simulink model "s2eig"  (Simulink 2.00)
settings: Solver=ode45  StartTime=0.0  StopTime=tstop  MaxStep=0.04  RelTol=1e-6  AbsTol=1e-6
values from neighbouring files (symbols this model uses):
  AEx = 0.0012    [I3ESSR.M]    (also in SET1.M)
  BEx = 1.264    [I3ESSR.M]    (also in SET1.M)
  delio = x(3)    [M1.M]    (also in M3.M = delta4; M3G.M = delta4; M4.M = delta)
  Domega = 0    [I3ESSR.M]    (also in M3.M; M3G.M; M5.M = 1; SET1.M = 2)
  Edpo = x(2)    [M1.M]    (also in M4.M = Vdo - xpq*Iqo + rs*Ido)
  Eqpo = x(1)    [M1.M]    (also in M4.M = Vqo + xpd*Ido + rs*Iqo)
  H = 2.89    [I3ESSR.M]    (also in M1.M = 0.5*J_rotor*wbasem*wbasem/Sbase; M3.M = diag(h); M3G.M = diag(h); M5.M = 0.352825293175)
  KA = 50    [I3ESSR.M]    (also in SET1.M)
  KE = -0.0465    [I3ESSR.M]    (also in SET1.M)
  KF = 0.0832    [I3ESSR.M]    (also in SET1.M)
  rs = 0.00    (= 0)    [I3ESSR.M]    (also in M1.M = rs/Zbase; M3.M; M3G.M = 0.001; M5.M = rs/Zb)
  TA = .06    (= 0.06)    [I3ESSR.M]    (also in SET1.M)
  TE = 0.052    [I3ESSR.M]    (also in SET1.M)
  TF = 1.0    (= 1)    [I3ESSR.M]    (also in SET1.M)
  Tpdo = 4.3    [I3ESSR.M]    (also in SET1.M = 7.9)
  Tpqo = 0.85    [I3ESSR.M]    (also in SET1.M = 0.41)
  VR = KE*Efo    [M4.M]
  VRmax = 1    [I3ESSR.M]    (also in SET1.M)
  VRmin = -1    [I3ESSR.M]    (also in SET1.M)
  Vs = Efo*KF/TF    [M4.M]
  wb = wbase    [M1.M]    (also in M2.M = 376.991118431; M3.M = 376.991118431; M3G.M = 376.991118431; M4.M = we)
  xd = 1.79    [I3ESSR.M]    (also in M1.M = xd/Zbase; M3.M; M3G.M; M5.M = xd/Zb)
  xpd = 0.169    [I3ESSR.M]    (also in M1.M = xpd/Zbase; SET1.M = 0.355)
  xq = 1.71    [I3ESSR.M]    (also in M1.M = xq/Zbase; M3.M; M3G.M; M5.M = xq/Zb)
undefined symbols (not defined in the file or in its folder): Ef, Exc_sw, Sbratio
settings Model: SaveTime=off  SaveOutput=off  ConsistencyChecking=off

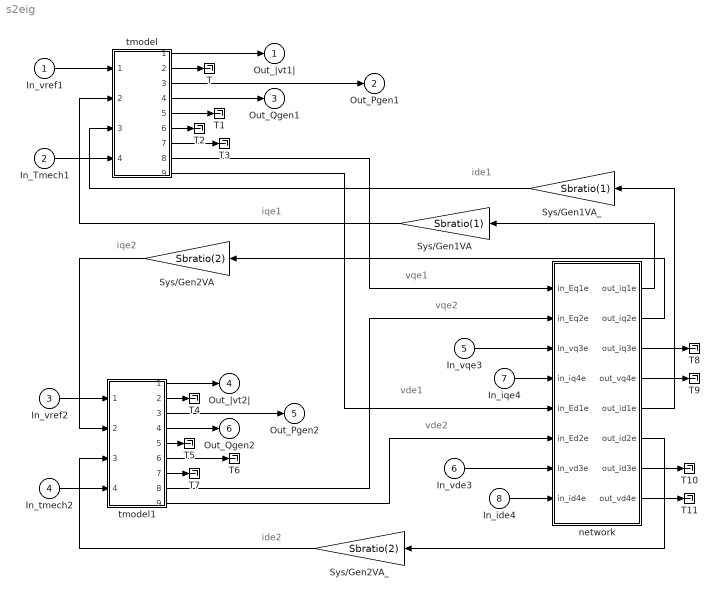
== system s2eig ==
  note: vqe1
  note: vqe2
  note: vde1
  note: vde2
  note: iqe2
  note: ide1
  note: iqe1
  note: ide2
  In_vref1 : Inport  Port=1  PortWidth=-1  SampleTime=-1
  In_Tmech1 : Inport  Port=2  PortWidth=-1  SampleTime=-1
  In_vref2 : Inport  Port=3  PortWidth=-1  SampleTime=-1
  In_tmech2 : Inport  Port=4  PortWidth=-1  SampleTime=-1
  In_vqe3 : Inport  Port=5  PortWidth=-1  SampleTime=-1
  In_vde3 : Inport  Port=6  PortWidth=-1  SampleTime=-1
  In_iqe4 : Inport  Port=7  PortWidth=-1  SampleTime=-1
  In_ide4 : Inport  Port=8  PortWidth=-1  SampleTime=-1
  Sys/Gen1VA : Gain  Orientation=left  Gain=Sbratio(1)
  Sys/Gen1VA_ : Gain  Orientation=left  Gain=Sbratio(1)
  Sys/Gen2VA : Gain  Orientation=left  Gain=Sbratio(2)
  Sys/Gen2VA_ : Gain  Orientation=left  Gain=Sbratio(2)
  T{,1..11} (12 alike) : Terminator
  network : Subsystem
  tmodel : Subsystem
  tmodel1 : Subsystem
  Out_|vt1| : Outport  Port=1  InitialOutput=0
  Out_Pgen1 : Outport  Port=2  InitialOutput=0
  Out_Qgen1 : Outport  Port=3  InitialOutput=0
  Out_|vt2| : Outport  Port=4  InitialOutput=0
  Out_Pgen2 : Outport  Port=5  InitialOutput=0
  Out_Qgen2 : Outport  Port=6  InitialOutput=0
  wires:
  network/4(out_vq4e) -> T9/1
  network/3(out_iq3e) -> T8/1
  network/8(out_vd4e) -> T11/1
  network/7(out_id3e) -> T10/1
  tmodel1/7(out_Tem) -> T7/1
  tmodel1/6(out_puslip) -> T6/1
  tmodel1/5(out_delta) -> T5/1
  tmodel1/2(out_|I|) -> T4/1
  tmodel/7(out_Tem) -> T3/1
  tmodel/6(out_puslip) -> T2/1
  tmodel/5(out_delta) -> T1/1
  tmodel/2(out_|I|) -> T/1
  Sys/Gen1VA/1 -> tmodel/2(in_iqe)
  network/1(out_iq1e) -> Sys/Gen1VA/1
  Sys/Gen1VA_/1 -> tmodel/3(in_ide)
  network/5(out_id1e) -> Sys/Gen1VA_/1
  Sys/Gen2VA_/1 -> tmodel1/3(in_ide)
  network/6(out_id2e) -> Sys/Gen2VA_/1
  Sys/Gen2VA/1 -> tmodel1/2(in_iqe)
  network/2(out_iq2e) -> Sys/Gen2VA/1
  tmodel1/4(out_Qgen) -> Out_Qgen2/1
  tmodel1/3(out_Pgen) -> Out_Pgen2/1
  tmodel1/1(out_|Vt|) -> Out_|vt2|/1
  tmodel/4(out_Qgen) -> Out_Qgen1/1
  tmodel/3(out_Pgen) -> Out_Pgen1/1
  tmodel/1(out_|Vt|) -> Out_|vt1|/1
  In_ide4/1 -> network/8(in_id4e)
  In_iqe4/1 -> network/4(in_iq4e)
  In_vde3/1 -> network/7(in_vd3e)
  In_vqe3/1 -> network/3(in_vq3e)
  In_tmech2/1 -> tmodel1/4(in_Tmech)
  In_vref2/1 -> tmodel1/1(in_Vref)
  In_Tmech1/1 -> tmodel/4(in_Tmech)
  In_vref1/1 -> tmodel/1(in_Vref)
  tmodel1/9(out_Edpe) -> network/6(in_Ed2e)
  tmodel/9(out_Edpe) -> network/5(in_Ed1e)
  tmodel1/8(out_Eqpe) -> network/2(in_Eq2e)
  tmodel/8(out_Eqpe) -> network/1(in_Eq1e)

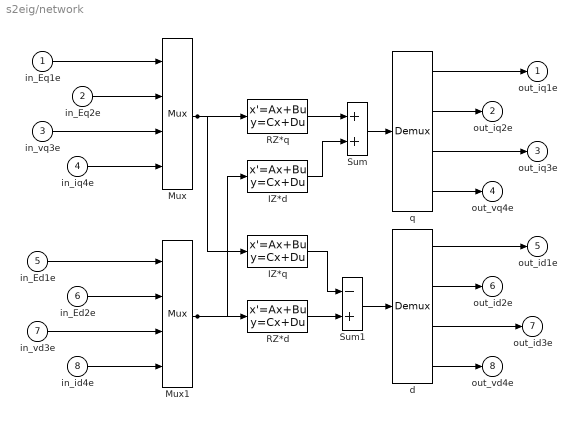
== system s2eig/network ==
  in_Eq1e : Inport  Port=1  PortWidth=-1  SampleTime=-1
  in_Eq2e : Inport  Port=2  PortWidth=-1  SampleTime=-1
  in_vq3e : Inport  Port=3  PortWidth=-1  SampleTime=-1
  in_iq4e : Inport  Port=4  PortWidth=-1  SampleTime=-1
  in_Ed1e : Inport  Port=5  PortWidth=-1  SampleTime=-1
  in_Ed2e : Inport  Port=6  PortWidth=-1  SampleTime=-1
  in_vd3e : Inport  Port=7  PortWidth=-1  SampleTime=-1
  in_id4e : Inport  Port=8  PortWidth=-1  SampleTime=-1
  IZ*d : StateSpace  A=[]  B=[]  C=[]  D=K  X0=0  mask(Matrix Gain){@1=IZ}
      mask prompts: @1 "Gain matrix:"
      mask help: Matrix Gain.
      mask init:
      | K = @1;
      mask Help: Multiplies input vector by entered matrix to produce output vector (y=Au).
      mask Display: disp('K')
  IZ*q : StateSpace  A=[]  B=[]  C=[]  D=K  X0=0  mask(Matrix Gain){@1=IZ}
      mask prompts: @1 "Gain matrix:"
      mask help: Matrix Gain.
      mask init:
      | K = @1;
      mask Help: Multiplies input vector by entered matrix to produce output vector (y=Au).
      mask Display: disp('K')
  Mux : Mux  Inputs=4
  Mux1 : Mux  Inputs=4
  RZ*d : StateSpace  A=[]  B=[]  C=[]  D=K  X0=0  mask(Matrix Gain){@1=RZ}
      mask prompts: @1 "Gain matrix:"
      mask help: Matrix Gain.
      mask init:
      | K = @1;
      mask Help: Multiplies input vector by entered matrix to produce output vector (y=Au).
      mask Display: disp('K')
  RZ*q : StateSpace  A=[]  B=[]  C=[]  D=K  X0=0  mask(Matrix Gain){@1=RZ}
      mask prompts: @1 "Gain matrix:"
      mask help: Matrix Gain.
      mask init:
      | K = @1;
      mask Help: Multiplies input vector by entered matrix to produce output vector (y=Au).
      mask Display: disp('K')
  Sum : Sum  Inputs=++
  Sum1 : Sum  Inputs=-+
  d : Demux  Outputs=4
  q : Demux  Outputs=4
  out_iq1e : Outport  Port=1  InitialOutput=0
  out_iq2e : Outport  Port=2  InitialOutput=0
  out_iq3e : Outport  Port=3  InitialOutput=0
  out_vq4e : Outport  Port=4  InitialOutput=0
  out_id1e : Outport  Port=5  InitialOutput=0
  out_id2e : Outport  Port=6  InitialOutput=0
  out_id3e : Outport  Port=7  InitialOutput=0
  out_vd4e : Outport  Port=8  InitialOutput=0
  wires:
  in_id4e/1 -> Mux1/4
  in_vd3e/1 -> Mux1/3
  in_Ed2e/1 -> Mux1/2
  in_Ed1e/1 -> Mux1/1
  in_iq4e/1 -> Mux/4
  in_vq3e/1 -> Mux/3
  in_Eq1e/1 -> Mux/1
  d/2 -> out_id2e/1
  d/4 -> out_vd4e/1
  d/3 -> out_id3e/1
  d/1 -> out_id1e/1
  q/2 -> out_iq2e/1
  in_Eq2e/1 -> Mux/2
  q/4 -> out_vq4e/1
  q/3 -> out_iq3e/1
  q/1 -> out_iq1e/1
  Mux/1 -> RZ*q/1, IZ*q/1
  Mux1/1 -> IZ*d/1, RZ*d/1
  RZ*q/1 -> Sum/1
  IZ*d/1 -> Sum/2
  IZ*q/1 -> Sum1/1
  RZ*d/1 -> Sum1/2
  Sum/1 -> q/1
  Sum1/1 -> d/1

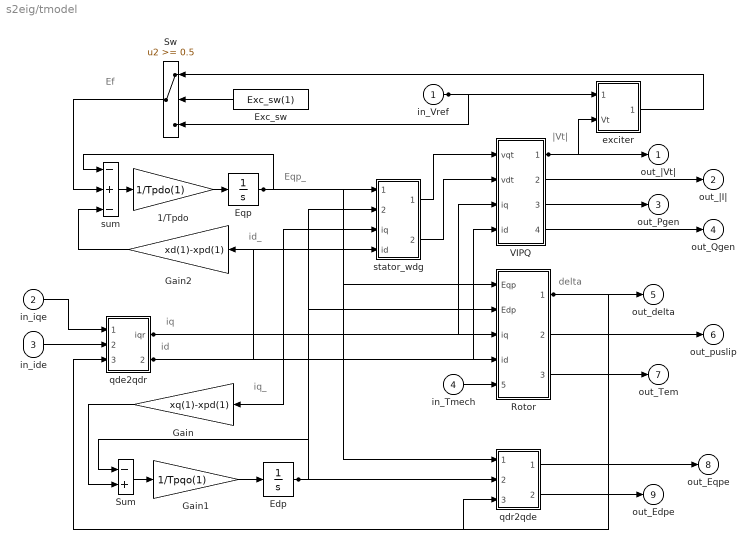
== system s2eig/tmodel ==
  note: iq_
  note: Ef
  note: delta
  note: id
  note: iq
  note: id_
  note: |Vt|
  note: Eqp_
  in_Vref : Inport  Port=1  PortWidth=-1  SampleTime=-1
  in_iqe : Inport  Port=2  PortWidth=-1  SampleTime=-1
  in_ide : Inport  Port=3  PortWidth=-1  SampleTime=-1
  in_Tmech : Inport  Port=4  PortWidth=-1  SampleTime=-1
  1/Tpdo : Gain  Gain=1/Tpdo(1)
  Edp : Integrator  ExternalReset=none  InitialConditionSource=internal  InitialCondition=Edpo(1)  LimitOutput=off  UpperSaturationLimit=inf  LowerSaturationLimit=-inf  ShowSaturationPort=off  ShowStatePort=off  AbsoluteTolerance=auto
  Eqp : Integrator  ExternalReset=none  InitialConditionSource=internal  InitialCondition=Eqpo(1)  LimitOutput=off  UpperSaturationLimit=inf  LowerSaturationLimit=-inf  ShowSaturationPort=off  ShowStatePort=off  AbsoluteTolerance=auto
  Exc_sw : Constant  Orientation=left  Value=Exc_sw(1)
  Gain : Gain  Orientation=left  Gain=xq(1)-xpd(1)
  Gain1 : Gain  Gain=1/Tpqo(1)
  Gain2 : Gain  Orientation=left  Gain=xd(1)-xpd(1)
  Rotor : Subsystem
  Sum : Sum  Inputs=-+
  Sw : Switch  Orientation=left  Threshold=0.5
  VIPQ : Subsystem
  exciter : Subsystem
  qde2qdr : Subsystem
  qdr2qde : Subsystem
  stator_wdg : Subsystem
  sum : Sum  Inputs=-+-
  out_|Vt| : Outport  Port=1  InitialOutput=0
  out_|I| : Outport  Port=2  InitialOutput=0
  out_Pgen : Outport  Port=3  InitialOutput=0
  out_Qgen : Outport  Port=4  InitialOutput=0
  out_delta : Outport  Port=5  InitialOutput=0
  out_puslip : Outport  Port=6  InitialOutput=0
  out_Tem : Outport  Port=7  InitialOutput=0
  out_Eqpe : Outport  Port=8  InitialOutput=0
  out_Edpe : Outport  Port=9  InitialOutput=0
  wires:
  in_Vref/1 -> Sw/3, exciter/1(Vref)
  stator_wdg/2(out_vdt) -> VIPQ/2(vdt)
  in_ide/1 -> qde2qdr/2(ide)
  qde2qdr/2(vdr) -> VIPQ/4(id), stator_wdg/4(id), Rotor/4(id), Gain2/1
  qde2qdr/1(iqr) -> VIPQ/3(iq), stator_wdg/3(iq), Rotor/3(iq), Gain/1
  Gain1/1 -> Edp/1
  Sum/1 -> Gain1/1
  Edp/1 -> qdr2qde/2(Edp), stator_wdg/2(Edp), Rotor/2(Edp), Sum/1
  Gain/1 -> Sum/2
  in_Tmech/1 -> Rotor/5(T_mech)
  qdr2qde/2(Edpe) -> out_Edpe/1
  qdr2qde/1(Eqpe) -> out_Eqpe/1
  VIPQ/1(out_|Vt|) -> out_|Vt|/1, exciter/2(Vt)
  stator_wdg/1(out_vqt) -> VIPQ/1(vqt)
  Rotor/3(Tem) -> out_Tem/1
  in_iqe/1 -> qde2qdr/1(iqe)
  Rotor/2(out_puslip) -> out_puslip/1
  Rotor/1(out_delta) -> qdr2qde/3(delta), out_delta/1, qde2qdr/3("delta ")
  VIPQ/4(out_Q) -> out_Qgen/1
  VIPQ/3(out_P) -> out_Pgen/1
  VIPQ/2(out_|I|) -> out_|I|/1
  Sw/1 -> sum/2
  Exc_sw/1 -> Sw/2
  exciter/1(out_Ef) -> Sw/1
  Gain2/1 -> sum/3
  sum/1 -> 1/Tpdo/1
  1/Tpdo/1 -> Eqp/1
  Eqp/1 -> qdr2qde/1(Eqp), sum/1, Rotor/1(Eqp), stator_wdg/1(Eqp)

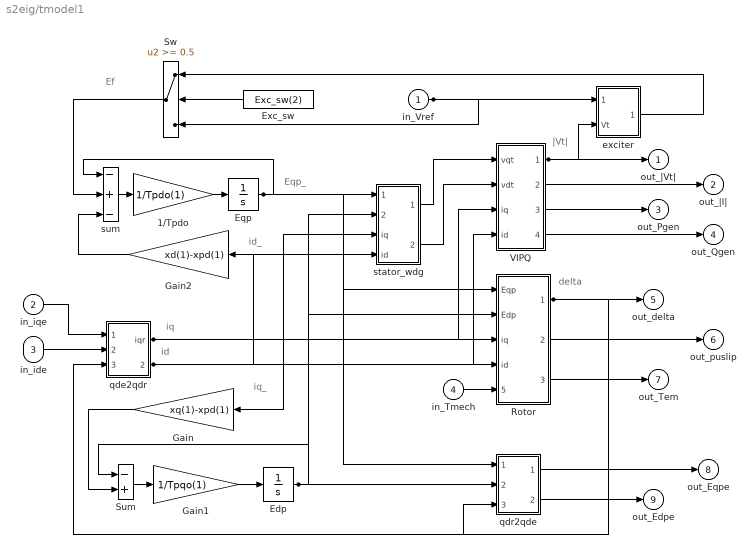
== system s2eig/tmodel1 ==
  note: id
  note: iq
  note: id_
  note: iq_
  note: delta
  note: Ef
  note: |Vt|
  note: Eqp_
  in_Vref : Inport  Port=1  PortWidth=-1  SampleTime=-1
  in_iqe : Inport  Port=2  PortWidth=-1  SampleTime=-1
  in_ide : Inport  Port=3  PortWidth=-1  SampleTime=-1
  in_Tmech : Inport  Port=4  PortWidth=-1  SampleTime=-1
  1/Tpdo : Gain  Gain=1/Tpdo(1)
  Edp : Integrator  ExternalReset=none  InitialConditionSource=internal  InitialCondition=Edpo(1)  LimitOutput=off  UpperSaturationLimit=inf  LowerSaturationLimit=-inf  ShowSaturationPort=off  ShowStatePort=off  AbsoluteTolerance=auto
  Eqp : Integrator  ExternalReset=none  InitialConditionSource=internal  InitialCondition=Eqpo(1)  LimitOutput=off  UpperSaturationLimit=inf  LowerSaturationLimit=-inf  ShowSaturationPort=off  ShowStatePort=off  AbsoluteTolerance=auto
  Exc_sw : Constant  Orientation=left  Value=Exc_sw(2)
  Gain : Gain  Orientation=left  Gain=xq(1)-xpd(1)
  Gain1 : Gain  Gain=1/Tpqo(1)
  Gain2 : Gain  Orientation=left  Gain=xd(1)-xpd(1)
  Rotor : Subsystem
  Sum : Sum  Inputs=-+
  Sw : Switch  Orientation=left  Threshold=0.5
  VIPQ : Subsystem
  exciter : Subsystem
  qde2qdr : Subsystem
  qdr2qde : Subsystem
  stator_wdg : Subsystem
  sum : Sum  Inputs=-+-
  out_|Vt| : Outport  Port=1  InitialOutput=0
  out_|I| : Outport  Port=2  InitialOutput=0
  out_Pgen : Outport  Port=3  InitialOutput=0
  out_Qgen : Outport  Port=4  InitialOutput=0
  out_delta : Outport  Port=5  InitialOutput=0
  out_puslip : Outport  Port=6  InitialOutput=0
  out_Tem : Outport  Port=7  InitialOutput=0
  out_Eqpe : Outport  Port=8  InitialOutput=0
  out_Edpe : Outport  Port=9  InitialOutput=0
  wires:
  in_Vref/1 -> Sw/3, exciter/1(Vref)
  stator_wdg/2(out_vdt) -> VIPQ/2(vdt)
  in_ide/1 -> qde2qdr/2(ide)
  qde2qdr/2(vdr) -> VIPQ/4(id), stator_wdg/4(id), Rotor/4(id), Gain2/1
  qde2qdr/1(iqr) -> VIPQ/3(iq), stator_wdg/3(iq), Rotor/3(iq), Gain/1
  Gain1/1 -> Edp/1
  Sum/1 -> Gain1/1
  Edp/1 -> qdr2qde/2(Edp), stator_wdg/2(Edp), Rotor/2(Edp), Sum/1
  Gain/1 -> Sum/2
  in_Tmech/1 -> Rotor/5(T_mech)
  qdr2qde/2(Edpe) -> out_Edpe/1
  qdr2qde/1(Eqpe) -> out_Eqpe/1
  VIPQ/1(out_|Vt|) -> out_|Vt|/1, exciter/2(Vt)
  stator_wdg/1(out_vqt) -> VIPQ/1(vqt)
  Rotor/3(Tem) -> out_Tem/1
  in_iqe/1 -> qde2qdr/1(iqe)
  Rotor/2(out_puslip) -> out_puslip/1
  Rotor/1(out_delta) -> qdr2qde/3(delta), out_delta/1, qde2qdr/3("delta ")
  VIPQ/4(out_Q) -> out_Qgen/1
  VIPQ/3(out_P) -> out_Pgen/1
  VIPQ/2(out_|I|) -> out_|I|/1
  Sw/1 -> sum/2
  Exc_sw/1 -> Sw/2
  exciter/1(out_Ef) -> Sw/1
  Gain2/1 -> sum/3
  sum/1 -> 1/Tpdo/1
  1/Tpdo/1 -> Eqp/1
  Eqp/1 -> qdr2qde/1(Eqp), sum/1, Rotor/1(Eqp), stator_wdg/1(Eqp)

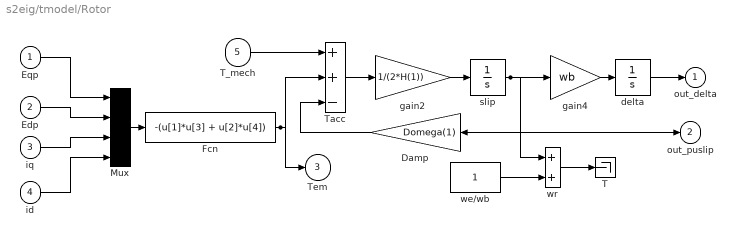
== system s2eig/tmodel/Rotor ==
  Eqp : Inport  Port=1  PortWidth=-1  SampleTime=-1
  Edp : Inport  Port=2  PortWidth=-1  SampleTime=-1
  iq : Inport  Port=3  PortWidth=-1  SampleTime=-1
  id : Inport  Port=4  PortWidth=-1  SampleTime=-1
  T_mech : Inport  Port=5  PortWidth=-1  SampleTime=-1
  Damp : Gain  Orientation=left  Gain=Domega(1)
  Fcn : Fcn  Expr=-(u[1]*u[3] + u[2]*u[4])
  Mux : Mux  Inputs=4
  T : Terminator
  Tacc : Sum  Inputs=++-
  delta : Integrator  ExternalReset=none  InitialConditionSource=internal  InitialCondition=delio(1)  LimitOutput=off  UpperSaturationLimit=inf  LowerSaturationLimit=-inf  ShowSaturationPort=off  ShowStatePort=off  AbsoluteTolerance=auto
  gain2 : Gain  Gain=1/(2*H(1))
  gain4 : Gain  Gain=wb
  slip : Integrator  ExternalReset=none  InitialConditionSource=internal  InitialCondition=0  LimitOutput=off  UpperSaturationLimit=inf  LowerSaturationLimit=-inf  ShowSaturationPort=off  ShowStatePort=off  AbsoluteTolerance=auto
  we/wb : Constant  Value=1
  wr : Sum  Inputs=++
  out_delta : Outport  Port=1  InitialOutput=0
  out_puslip : Outport  Port=2  InitialOutput=0
  Tem : Outport  Port=3  InitialOutput=0
  wires:
  wr/1 -> T/1
  Tacc/1 -> gain2/1
  id/1 -> Mux/4
  iq/1 -> Mux/3
  Fcn/1 -> Tem/1, Tacc/2
  Mux/1 -> Fcn/1
  Eqp/1 -> Mux/1
  Edp/1 -> Mux/2
  slip/1 -> Damp/1, gain4/1, out_puslip/1, wr/1
  gain4/1 -> delta/1
  gain2/1 -> slip/1
  we/wb/1 -> wr/2
  delta/1 -> out_delta/1
  T_mech/1 -> Tacc/1
  Damp/1 -> Tacc/3

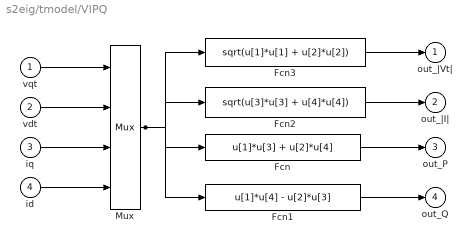
== system s2eig/tmodel/VIPQ ==
  vqt : Inport  Port=1  PortWidth=-1  SampleTime=-1
  vdt : Inport  Port=2  PortWidth=-1  SampleTime=-1
  iq : Inport  Port=3  PortWidth=-1  SampleTime=-1
  id : Inport  Port=4  PortWidth=-1  SampleTime=-1
  Fcn : Fcn  Expr=u[1]*u[3] + u[2]*u[4]
  Fcn1 : Fcn  Expr=u[1]*u[4] - u[2]*u[3]
  Fcn2 : Fcn  Expr=sqrt(u[3]*u[3] + u[4]*u[4])
  Fcn3 : Fcn  Expr=sqrt(u[1]*u[1] + u[2]*u[2])
  Mux : Mux  Inputs=4
  out_|Vt| : Outport  Port=1  InitialOutput=0
  out_|I| : Outport  Port=2  InitialOutput=0
  out_P : Outport  Port=3  InitialOutput=0
  out_Q : Outport  Port=4  InitialOutput=0
  wires:
  iq/1 -> Mux/3
  vdt/1 -> Mux/2
  Fcn2/1 -> out_|I|/1
  Fcn3/1 -> out_|Vt|/1
  Mux/1 -> Fcn2/1, Fcn3/1, Fcn1/1, Fcn/1
  Fcn1/1 -> out_Q/1
  Fcn/1 -> out_P/1
  id/1 -> Mux/4
  vqt/1 -> Mux/1

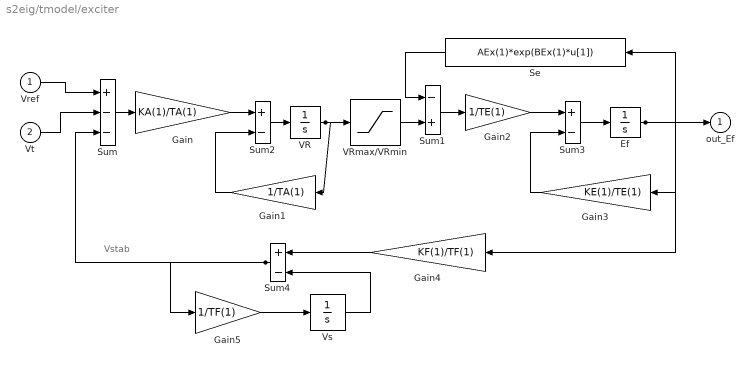
== system s2eig/tmodel/exciter ==
  note: Vstab
  Vref : Inport  Port=1  PortWidth=-1  SampleTime=-1
  Vt : Inport  Port=2  PortWidth=-1  SampleTime=-1
  Ef : Integrator  ExternalReset=none  InitialConditionSource=internal  InitialCondition=Ef(1)  LimitOutput=off  UpperSaturationLimit=inf  LowerSaturationLimit=-inf  ShowSaturationPort=off  ShowStatePort=off  AbsoluteTolerance=auto
  Gain : Gain  Gain=KA(1)/TA(1)
  Gain1 : Gain  Orientation=left  Gain=1/TA(1)
  Gain2 : Gain  Gain=1/TE(1)
  Gain3 : Gain  Orientation=left  Gain=KE(1)/TE(1)
  Gain4 : Gain  Orientation=left  Gain=KF(1)/TF(1)
  Gain5 : Gain  Gain=1/TF(1)
  Se : Fcn  Orientation=left  Expr=AEx(1)*exp(BEx(1)*u[1])
  Sum : Sum  Inputs=+--
  Sum1 : Sum  Inputs=-+
  Sum2 : Sum  Inputs=+-
  Sum3 : Sum  Inputs=+-
  Sum4 : Sum  Orientation=left  Inputs=+-
  VR : Integrator  ExternalReset=none  InitialConditionSource=internal  InitialCondition=VR(1)  LimitOutput=off  UpperSaturationLimit=inf  LowerSaturationLimit=-inf  ShowSaturationPort=off  ShowStatePort=off  AbsoluteTolerance=auto
  VRmax/VRmin : Saturate  UpperLimit=VRmax(1)  LowerLimit=VRmin(1)
  Vs : Integrator  ExternalReset=none  InitialConditionSource=internal  InitialCondition=Vs(1)  LimitOutput=off  UpperSaturationLimit=inf  LowerSaturationLimit=-inf  ShowSaturationPort=off  ShowStatePort=off  AbsoluteTolerance=auto
  out_Ef : Outport  Port=1  InitialOutput=0
  wires:
  Sum4/1 -> Gain5/1, Sum/3
  Vs/1 -> Sum4/2
  Gain5/1 -> Vs/1
  Gain4/1 -> Sum4/1
  Gain1/1 -> Sum2/2
  Gain/1 -> Sum2/1
  Ef/1 -> Gain4/1, out_Ef/1, Se/1, Gain3/1
  Gain3/1 -> Sum3/2
  Gain2/1 -> Sum3/1
  Sum1/1 -> Gain2/1
  Sum3/1 -> Ef/1
  VR/1 -> Gain1/1, VRmax/VRmin/1
  Sum/1 -> Gain/1
  Sum2/1 -> VR/1
  Se/1 -> Sum1/1
  Vref/1 -> Sum/1
  VRmax/VRmin/1 -> Sum1/2
  Vt/1 -> Sum/2

== system s2eig/tmodel/qde2qdr ==
  iqe : Inport  Port=1  PortWidth=-1  SampleTime=-1
  ide : Inport  Port=2  PortWidth=-1  SampleTime=-1
  "delta " : Inport  Port=3  PortWidth=-1  SampleTime=-1
  Mux : Mux  Inputs=3
  fcn : Fcn  Expr=u[1]*cos(u[3]) - u[2]*sin(u[3])
  fcn1 : Fcn  Expr=u[1]*sin(u[3]) + u[2]*cos(u[3])
  iqr : Outport  Port=1  InitialOutput=0
  vdr : Outport  Port=2  InitialOutput=0
  wires:
  ide/1 -> Mux/2
  "delta "/1 -> Mux/3
  Mux/1 -> fcn1/1, fcn/1
  fcn/1 -> iqr/1
  iqe/1 -> Mux/1
  fcn1/1 -> vdr/1

== system s2eig/tmodel/qdr2qde ==
  Eqp : Inport  Port=1  PortWidth=-1  SampleTime=-1
  Edp : Inport  Port=2  PortWidth=-1  SampleTime=-1
  delta : Inport  Port=3  PortWidth=-1  SampleTime=-1
  Mux : Mux  Inputs=3
  fcn : Fcn  Expr=u[1]*cos(u[3]) + u[2]*sin(u[3])
  fcn1 : Fcn  Expr=-u[1]*sin(u[3]) + u[2]*cos(u[3])
  Eqpe : Outport  Port=1  InitialOutput=0
  Edpe : Outport  Port=2  InitialOutput=0
  wires:
  delta/1 -> Mux/3
  Edp/1 -> Mux/2
  Mux/1 -> fcn1/1, fcn/1
  fcn/1 -> Eqpe/1
  Eqp/1 -> Mux/1
  fcn1/1 -> Edpe/1

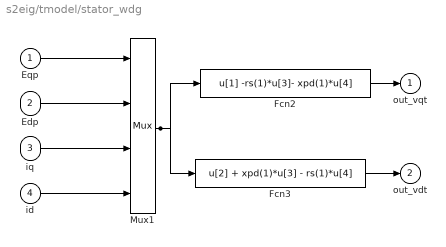
== system s2eig/tmodel/stator_wdg ==
  Eqp : Inport  Port=1  PortWidth=-1  SampleTime=-1
  Edp : Inport  Port=2  PortWidth=-1  SampleTime=-1
  iq : Inport  Port=3  PortWidth=-1  SampleTime=-1
  id : Inport  Port=4  PortWidth=-1  SampleTime=-1
  Fcn2 : Fcn  Expr=u[1] -rs(1)*u[3]- xpd(1)*u[4]
  Fcn3 : Fcn  Expr=u[2] + xpd(1)*u[3] - rs(1)*u[4]
  Mux1 : Mux  Inputs=4
  out_vqt : Outport  Port=1  InitialOutput=0
  out_vdt : Outport  Port=2  InitialOutput=0
  wires:
  Edp/1 -> Mux1/2
  id/1 -> Mux1/4
  iq/1 -> Mux1/3
  Fcn3/1 -> out_vdt/1
  Fcn2/1 -> out_vqt/1
  Mux1/1 -> Fcn3/1, Fcn2/1
  Eqp/1 -> Mux1/1

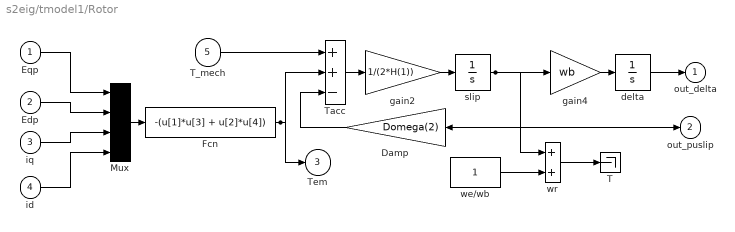
== system s2eig/tmodel1/Rotor ==
  Eqp : Inport  Port=1  PortWidth=-1  SampleTime=-1
  Edp : Inport  Port=2  PortWidth=-1  SampleTime=-1
  iq : Inport  Port=3  PortWidth=-1  SampleTime=-1
  id : Inport  Port=4  PortWidth=-1  SampleTime=-1
  T_mech : Inport  Port=5  PortWidth=-1  SampleTime=-1
  Damp : Gain  Orientation=left  Gain=Domega(2)
  Fcn : Fcn  Expr=-(u[1]*u[3] + u[2]*u[4])
  Mux : Mux  Inputs=4
  T : Terminator
  Tacc : Sum  Inputs=++-
  delta : Integrator  ExternalReset=none  InitialConditionSource=internal  InitialCondition=delio(1)  LimitOutput=off  UpperSaturationLimit=inf  LowerSaturationLimit=-inf  ShowSaturationPort=off  ShowStatePort=off  AbsoluteTolerance=auto
  gain2 : Gain  Gain=1/(2*H(1))
  gain4 : Gain  Gain=wb
  slip : Integrator  ExternalReset=none  InitialConditionSource=internal  InitialCondition=0  LimitOutput=off  UpperSaturationLimit=inf  LowerSaturationLimit=-inf  ShowSaturationPort=off  ShowStatePort=off  AbsoluteTolerance=auto
  we/wb : Constant  Value=1
  wr : Sum  Inputs=++
  out_delta : Outport  Port=1  InitialOutput=0
  out_puslip : Outport  Port=2  InitialOutput=0
  Tem : Outport  Port=3  InitialOutput=0
  wires:
  wr/1 -> T/1
  Tacc/1 -> gain2/1
  id/1 -> Mux/4
  iq/1 -> Mux/3
  Fcn/1 -> Tem/1, Tacc/2
  Mux/1 -> Fcn/1
  Eqp/1 -> Mux/1
  Edp/1 -> Mux/2
  slip/1 -> Damp/1, gain4/1, out_puslip/1, wr/1
  gain4/1 -> delta/1
  gain2/1 -> slip/1
  we/wb/1 -> wr/2
  delta/1 -> out_delta/1
  T_mech/1 -> Tacc/1
  Damp/1 -> Tacc/3

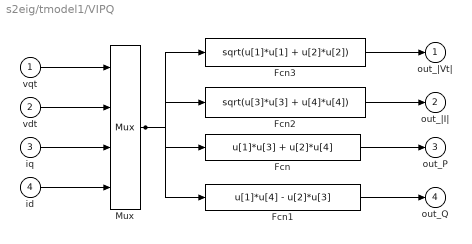
== system s2eig/tmodel1/VIPQ ==
  vqt : Inport  Port=1  PortWidth=-1  SampleTime=-1
  vdt : Inport  Port=2  PortWidth=-1  SampleTime=-1
  iq : Inport  Port=3  PortWidth=-1  SampleTime=-1
  id : Inport  Port=4  PortWidth=-1  SampleTime=-1
  Fcn : Fcn  Expr=u[1]*u[3] + u[2]*u[4]
  Fcn1 : Fcn  Expr=u[1]*u[4] - u[2]*u[3]
  Fcn2 : Fcn  Expr=sqrt(u[3]*u[3] + u[4]*u[4])
  Fcn3 : Fcn  Expr=sqrt(u[1]*u[1] + u[2]*u[2])
  Mux : Mux  Inputs=4
  out_|Vt| : Outport  Port=1  InitialOutput=0
  out_|I| : Outport  Port=2  InitialOutput=0
  out_P : Outport  Port=3  InitialOutput=0
  out_Q : Outport  Port=4  InitialOutput=0
  wires:
  iq/1 -> Mux/3
  vdt/1 -> Mux/2
  Fcn2/1 -> out_|I|/1
  Fcn3/1 -> out_|Vt|/1
  Mux/1 -> Fcn2/1, Fcn3/1, Fcn1/1, Fcn/1
  Fcn1/1 -> out_Q/1
  Fcn/1 -> out_P/1
  id/1 -> Mux/4
  vqt/1 -> Mux/1

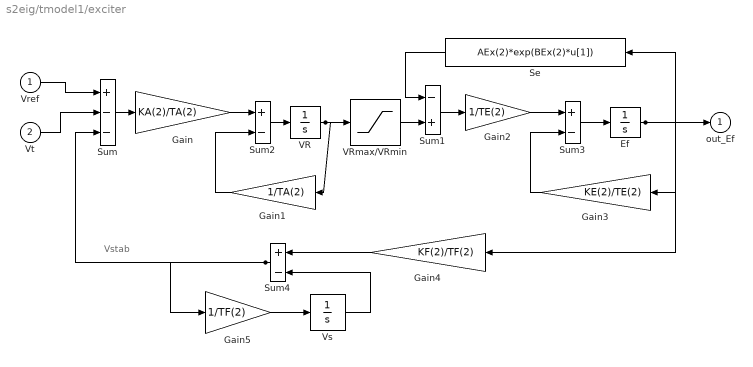
== system s2eig/tmodel1/exciter ==
  note: Vstab
  Vref : Inport  Port=1  PortWidth=-1  SampleTime=-1
  Vt : Inport  Port=2  PortWidth=-1  SampleTime=-1
  Ef : Integrator  ExternalReset=none  InitialConditionSource=internal  InitialCondition=Ef(2)  LimitOutput=off  UpperSaturationLimit=inf  LowerSaturationLimit=-inf  ShowSaturationPort=off  ShowStatePort=off  AbsoluteTolerance=auto
  Gain : Gain  Gain=KA(2)/TA(2)
  Gain1 : Gain  Orientation=left  Gain=1/TA(2)
  Gain2 : Gain  Gain=1/TE(2)
  Gain3 : Gain  Orientation=left  Gain=KE(2)/TE(2)
  Gain4 : Gain  Orientation=left  Gain=KF(2)/TF(2)
  Gain5 : Gain  Gain=1/TF(2)
  Se : Fcn  Orientation=left  Expr=AEx(2)*exp(BEx(2)*u[1])
  Sum : Sum  Inputs=+--
  Sum1 : Sum  Inputs=-+
  Sum2 : Sum  Inputs=+-
  Sum3 : Sum  Inputs=+-
  Sum4 : Sum  Orientation=left  Inputs=+-
  VR : Integrator  ExternalReset=none  InitialConditionSource=internal  InitialCondition=VR(2)  LimitOutput=off  UpperSaturationLimit=inf  LowerSaturationLimit=-inf  ShowSaturationPort=off  ShowStatePort=off  AbsoluteTolerance=auto
  VRmax/VRmin : Saturate  UpperLimit=VRmax(2)  LowerLimit=VRmin(2)
  Vs : Integrator  ExternalReset=none  InitialConditionSource=internal  InitialCondition=Vs(2)  LimitOutput=off  UpperSaturationLimit=inf  LowerSaturationLimit=-inf  ShowSaturationPort=off  ShowStatePort=off  AbsoluteTolerance=auto
  out_Ef : Outport  Port=1  InitialOutput=0
  wires:
  Sum4/1 -> Gain5/1, Sum/3
  Vs/1 -> Sum4/2
  Gain5/1 -> Vs/1
  Gain4/1 -> Sum4/1
  Gain1/1 -> Sum2/2
  Gain/1 -> Sum2/1
  Ef/1 -> Gain4/1, out_Ef/1, Se/1, Gain3/1
  Gain3/1 -> Sum3/2
  Gain2/1 -> Sum3/1
  Sum1/1 -> Gain2/1
  Sum3/1 -> Ef/1
  VR/1 -> Gain1/1, VRmax/VRmin/1
  Sum/1 -> Gain/1
  Sum2/1 -> VR/1
  Se/1 -> Sum1/1
  Vref/1 -> Sum/1
  VRmax/VRmin/1 -> Sum1/2
  Vt/1 -> Sum/2

== system s2eig/tmodel1/qde2qdr ==
  iqe : Inport  Port=1  PortWidth=-1  SampleTime=-1
  ide : Inport  Port=2  PortWidth=-1  SampleTime=-1
  "delta " : Inport  Port=3  PortWidth=-1  SampleTime=-1
  Mux : Mux  Inputs=3
  fcn : Fcn  Expr=u[1]*cos(u[3]) - u[2]*sin(u[3])
  fcn1 : Fcn  Expr=u[1]*sin(u[3]) + u[2]*cos(u[3])
  iqr : Outport  Port=1  InitialOutput=0
  vdr : Outport  Port=2  InitialOutput=0
  wires:
  ide/1 -> Mux/2
  "delta "/1 -> Mux/3
  Mux/1 -> fcn1/1, fcn/1
  fcn/1 -> iqr/1
  iqe/1 -> Mux/1
  fcn1/1 -> vdr/1

== system s2eig/tmodel1/qdr2qde ==
  Eqp : Inport  Port=1  PortWidth=-1  SampleTime=-1
  Edp : Inport  Port=2  PortWidth=-1  SampleTime=-1
  delta : Inport  Port=3  PortWidth=-1  SampleTime=-1
  Mux : Mux  Inputs=3
  fcn : Fcn  Expr=u[1]*cos(u[3]) + u[2]*sin(u[3])
  fcn1 : Fcn  Expr=-u[1]*sin(u[3]) + u[2]*cos(u[3])
  Eqpe : Outport  Port=1  InitialOutput=0
  Edpe : Outport  Port=2  InitialOutput=0
  wires:
  delta/1 -> Mux/3
  Edp/1 -> Mux/2
  Mux/1 -> fcn1/1, fcn/1
  fcn/1 -> Eqpe/1
  Eqp/1 -> Mux/1
  fcn1/1 -> Edpe/1

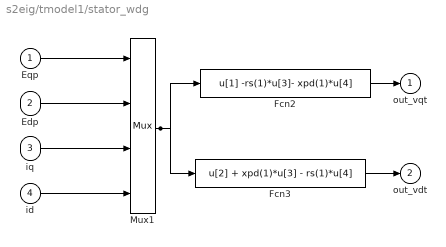
== system s2eig/tmodel1/stator_wdg ==
  Eqp : Inport  Port=1  PortWidth=-1  SampleTime=-1
  Edp : Inport  Port=2  PortWidth=-1  SampleTime=-1
  iq : Inport  Port=3  PortWidth=-1  SampleTime=-1
  id : Inport  Port=4  PortWidth=-1  SampleTime=-1
  Fcn2 : Fcn  Expr=u[1] -rs(1)*u[3]- xpd(1)*u[4]
  Fcn3 : Fcn  Expr=u[2] + xpd(1)*u[3] - rs(1)*u[4]
  Mux1 : Mux  Inputs=4
  out_vqt : Outport  Port=1  InitialOutput=0
  out_vdt : Outport  Port=2  InitialOutput=0
  wires:
  Edp/1 -> Mux1/2
  id/1 -> Mux1/4
  iq/1 -> Mux1/3
  Fcn3/1 -> out_vdt/1
  Fcn2/1 -> out_vqt/1
  Mux1/1 -> Fcn3/1, Fcn2/1
  Eqp/1 -> Mux1/1
